simulink model "generic_IsaacV5_Werkend_Clean"  (R2015a)
settings: Solver=ode45  StartTime=0.0  StopTime=inf  FixedStep=0.001  RelTol=1e-3
model workspace (MAT data in the model file):
  Gr = 10.32
  H = 0.2735
  Krf_a = 183.26
  Krr_a = 325.31
  Ksf = 12153
  Ksr = 14563
  Kwf = 0
  Kwr = 0
  L = 1.525
  Lf = 0.78
  Lr = 0.745
  M = 265
  Reff = 0.2325
  Sr = 0.6
  Tf = 1.2
  Tmax = 40
  Tr = 1.2
  g = 9.81
  mu_max = 1.5
libraries: CarMaker4SL x22, simulink x1
(part 3 of 3)

== matlab function generic_IsaacV5_Werkend_Clean/CarMaker/TorqueVectoring/Post-processor/Slip-controle  ==
  data: ax input; ay input; mu_max input; A output; Vzwp input; B output; C output; D output; Wf output; Wr output
function [A,B,C,D,Wf,Wr] = Slip_controle(ax,ay,mu_max,Vzwp)
% Berekening van de maximale torques die men kan toepassen op de wielen
% door berekening van de normaalkrachten op de wielen.

%load('parameters.mat');

M       = 265;             
L       = 1.525;                           
Lf      = 0.780;                              
Lr      = 0.745;                              
Tf      = 1.200;                             
Tr      = 1.200;                            
g       = 9.81;                                                       
Krf_a	= 183.26;                            
Krr_a	= 325.31;                           
Ksf     = 12153;             %Veerstijfheid vooraan
Ksr     = 14563;
H       = 0.2735;                        
    %ax      =0;                 
    %ay      =0;                               
    %Vzwp    =0;                 
    %mu_max  =1.5;

%Wielbelastingen

%Statische wielbelasting
Ws_fl = ((Lr*M*g)/(2*L));
Ws_fr = ((Lr*M*g)/(2*L));
Ws_rl = ((Lf*M*g)/(2*L));
Ws_rr = ((Lf*M*g)/(2*L));

%Ws_f = Ws_fl + Ws_fr;
%Ws_r = Ws_rl + Ws_rr;

%Laterale wielbelasting (door rollen van de wagen)
Wy_fl = -((H*M*ay)/(2*Tf));                         %Kracht per wiel
Wy_fr =  ((H*M*ay)/(2*Tf));
Wy_rl = -((H*M*ay)/(2*Tr));
Wy_rr =  ((H*M*ay)/(2*Tr));

%Longitudinale wielbelasting
Wx_fl = -((H*M*ax)/(2*L));                          %Kracht per wiel
Wx_fr = -((H*M*ax)/(2*L));
Wx_rl =  ((H*M*ax)/(2*L));
Wx_rr =  ((H*M*ax)/(2*L));

%Aerodynamische wielbelasting
LF = -0.0237*(Vzwp)^2 + 0.0958*Vzwp;                %Nog na te kijken; komt uit excel van aeromannen
LR = -0.0237*(Vzwp)^2 + 0.0958*Vzwp;                %Nog na te kijken; komt uit excel van aeromannen

Wa_fl = (-LF/2);  %+((Krf/(Krf+Krr))*(Rm/Tf));      %is er hier 2x rolmoment??? (zie lateraal)
Wa_fr = (-LF/2);  %-((Krf/(Krf+Krr))*(Rm/Tf));
Wa_rl = (-LR/2);  %+((Krr/(Krf+Krr))*(Rm/Tr));
Wa_rr = (-LR/2);  %-((Krr/(Krf+Krr))*(Rm/Tr));

%anti-roll bar wielbelasting
Wab_fl =  ((Krf_a*(-Wy_fl))/((Krf_a+((Ksf*(Tf)^2)/2))));
Wab_fr =  ((Krf_a*(-Wy_fr))/((Krf_a+((Ksf*(Tf)^2)/2))));
Wab_rl =  ((Krr_a*(-Wy_rl))/((Krr_a+((Ksr*(Tr)^2)/2))));
Wab_rr =  ((Krr_a*(-Wy_rr))/((Krr_a+((Ksr*(Tr)^2)/2))));

%Totale belasting per wiel
Wfl = Ws_fl + Wy_fl + Wx_fl + Wa_fl + Wab_fl;   %Ongebruikt, kan later eventueel gebruikt worden voor 4WD??
Wfr = Ws_fr + Wy_fr + Wx_fr + Wa_fr + Wab_fr;   %^ Idem
Wrl = Ws_rl + Wy_rl + Wx_rl + Wa_rl + Wab_rl;
Wrr = Ws_rr + Wy_rr + Wx_rr + Wa_rr + Wab_rr;



%%Omrekening naar torques
%HIER GEWIJZIGD

%Wrijvingscirkels (wortels worden naar buiten gebracht; kunnen niet
%berekend worden in code; geeft fouten; vervolgens ook vermenigvuldigen 
%met effectieve bandenstraal om tot de wielkoppels te komen)

%Jx_rl = ((Wrl*mu_max)^2-((Wrl*ay)/(g))^2);
%Jx_rr = ((Wrr*mu_max)^2-((Wrr*ay)/(g))^2);

%     if Jx_rl < 0
%     then Jx_rl = 0
% end
% 
% if Jx_rr < 0
%     then Jx_rr = 0
% end


A = (Wrl*mu_max)^2;
B = ((Wrl*ay)/(g))^2;
C = (Wrr*mu_max)^2;
D = ((Wrr*ay)/(g))^2;

% Fx_rl = sqrt((Wrl*mu_max)^2-((Wrl*ay)/(g))^2);
% 
% Fx_rr = sqrt((Wrr*mu_max)^2-((Wrr*ay)/(g))^2);

%Maximum torques
% Trl_max = Fx_rl*Reff;
% Trr_max = Fx_rr*Reff;

%Belastingen per as
Wf = (Wfl+Wfr)/2;
Wr = (Wrl+Wrr)/2;

== matlab function generic_IsaacV5_Werkend_Clean/CarMaker/TorqueVectoring/Pre-processor/prepros - code/Pre-processor ==
  data: Yaw_ref output; Vzwp input; stuurhoek input; mu_max input; a_zwpx input; Fy_f input; Fy_r input; alfa_r1 input; alfa_f output; alfa_r output; alfa_f1 input
function [Yaw_ref,alfa_f,alfa_r]= pre_processor(Vzwp,stuurhoek,mu_max,a_zwpx,Fy_f,Fy_r,alfa_r1,alfa_f1)
%De pre-processor berekend de gewenste yaw rate door het minimum te nemen
%van de ideale en de maximale yaw rate waarde.
%Belangrijk hierbij de hoeken in RAD!!!!!!

%Parameters
M       = 265;             
L       = 1.525;                           
Lf      = 0.780;                              
Lr      = 0.745; 
g       = 9.81;

%Berekening massa's
Wf = (M*Lr*g/L);
Wr = (M*Lf*g/L);

% berekening van de sliphoek beita
beita = atan(Lf * tan(stuurhoek)/ (Lf+Lr)) ;



%Berekening Cornering stiffness
               Cf = (Fy_f/alfa_f1);
               Cr = (Fy_r/alfa_r1);
%              C_rl = (Fy_rl/alfa_rl);
%              C_rr = (Fy_rr/alfa_rr);
                
 % Fy_f = Cf * alfa_f ;
 % Fy_r = Cr * alfa_r ;
%Gemiddelde van de cornering stiffness vooraan en achteraan nemen
          %Cf = ((C_fl + C_fr)/ 2);
          %Cr = ((C_rl + C_rr)/ 2);
%Berekening van de onderstuur factor.
Ku = ((Wf/Cf)-(Wr/Cr));

%Berekening van de ideale yaw rate.
Yaw_id = ((Vzwp*stuurhoek)/((Lf+Lr)+Ku*(Vzwp)^2));

%Berekening van de maximale yaw rate.
Yaw_max = (((mu_max*g)-(a_zwpx * tan(beita)) - (Vzwp * cos(beita)* diff(beita)))/(Vzwp*cos(beita)));

%Minimale yaw rate.
Yaw_ref = min([Yaw_id ; Yaw_max]);
%Berekening sliphoeken
alfa_f = - beita + stuurhoek - ((Lf * Yaw_ref)/Vzwp);
alfa_r = - beita + ((Lr * Yaw_ref)/Vzwp);
